simulink model "kepler_basic_2021b"  (R2021b)
settings: Solver=ode4  StartTime=0.0  StopTime=6000  FixedStep=0.01  RelTol=1e-3
(part 1 of 2)
settings Model: Creator=sakur  LastModifiedBy=sakur
settings DebuggingCC: UnconnectedInputMsg=none  UnconnectedOutputMsg=none  UnconnectedLineMsg=none
settings RTWCC: DLArmComputeVersion=20.02.1

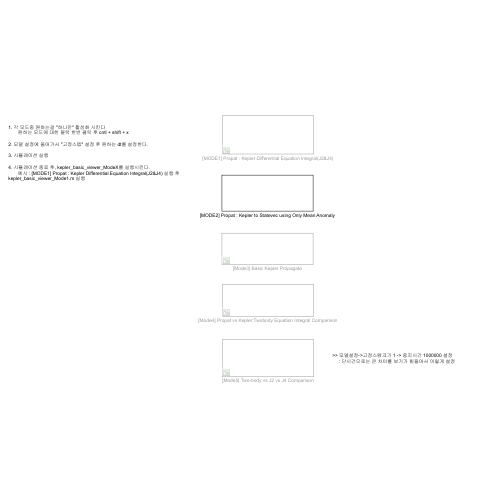
[thumbnail: Simulink's stored preview of the top-level diagram]
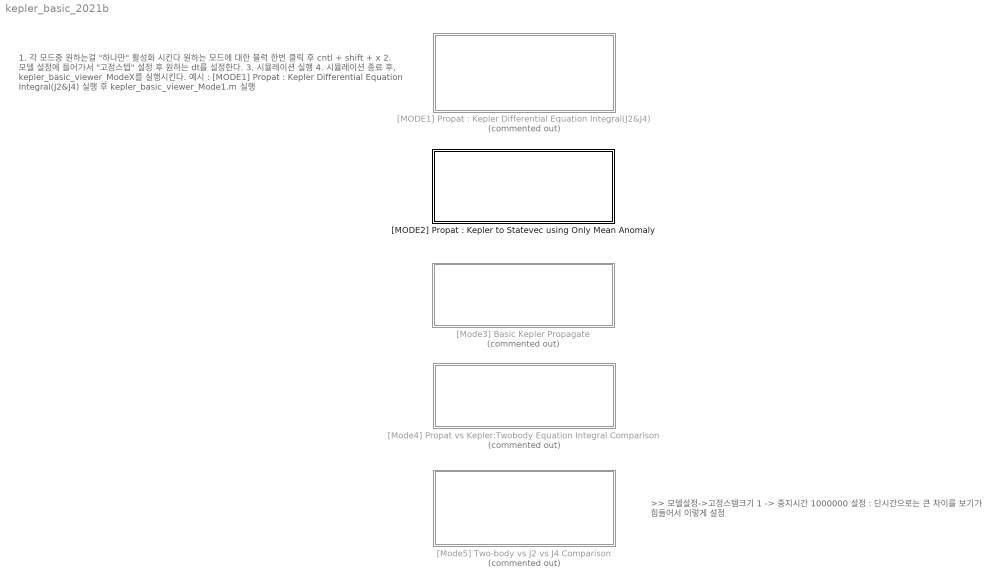
== system kepler_basic_2021b ==
  note: >> 모델설정->고정스템크기 1 -> 중지시간 1000000 설정
      |      : 단시간으로는 큰 차이를 보기가 힘들어서 이렇게 설정
  note: 1. 각 모드중 원하는걸 "하나만" 활성화 시킨다
      | 	원하는 모드에 대한 블럭 한번 클릭 후 cntl + shift + x
      |
      | 2. 모델 설정에 들어가서 "고정스텝" 설정 후 원하는 dt를 설정한다.
      |
      | 3. 시뮬레이션 실행
      |
      | 4. 시뮬레이션 종료 후, kepler_basic_viewer_ModeX를 실행시킨다.
      | 	예시 : [MODE1] Propat : Kepler Differential Equation Integral(J2&J4) 실행 후 kepler_basic_viewer_Mode1.m 실행
  "[MODE1] Propat : Kepler Differential Equation Integral(J2&J4)" : Subsystem  Commented=on
  "[MODE2] Propat : Kepler to Statevec using Only Mean Anomaly" : Subsystem
  "[Mode3] Basic Kepler Propagate" : Subsystem  Commented=on
  "[Mode4] Propat vs Kepler:Twobody Equation Integral Comparison" : Subsystem  Commented=on
  "[Mode5] Two-body vs J2 vs J4 Comparison" : Subsystem  Commented=on

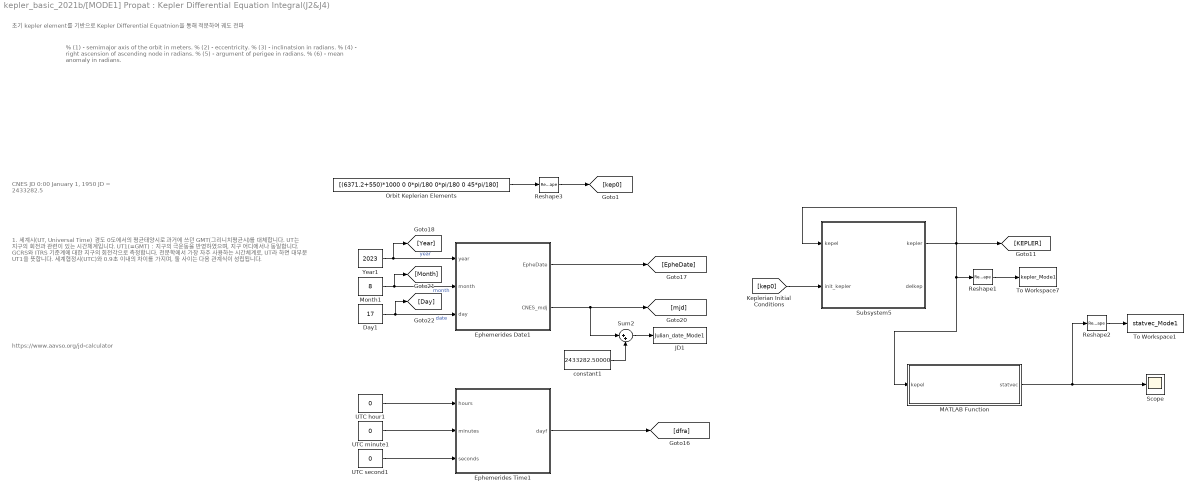
== system kepler_basic_2021b/[MODE1] Propat : Kepler Differential Equation Integral(J2&J4) ==
  note: 초기 kepler element를 기반으로 Kepler Differential Equatnion을 통해 적분하여 궤도 전파
  note: CNES JD
      | 0:00 January 1, 1950
      | JD − 2433282.5
  note: https://www.aavso.org/jd-calculator
  note: 1. 세계시(UT, Universal Time)
      | 경도 0도에서의 평균태양시로 과거에 쓰던 GMT(그리니치평균시)를 대체합니다. UT는 지구의 회전과 관련이 있는 시간체계입니다.
      |
      | UT1(=GMT) : 지구의 극운동을 반영하였으며, 지구 어디에서나 동일합니다. GCRS와 ITRS 기준계에 대한 지구의 회전각으로 측정합니다. 천문학에서 가장 자주 사용하는 시간체계로, UT라 하면 대부분 UT1을 뜻합니다. 세계협정시(UTC)와 0.9초 이내의 차이를 가지며, 둘 사이는 다음 관계식이 성립됩니다.
  note: % (1) - semimajor axis of the orbit in meters.
      | % (2) - eccentricity.
      | % (3) - inclinatsion in radians.
      | % (4) - right ascension of ascending node in radians.
      | % (5) - argument of perigee in radians.
      | % (6) - mean anomaly in radians.
  Day1 : Constant  Value=17
  Ephemerides Date1 : Subsystem
  Ephemerides Time1 : MATLAB Function  TreatAsAtomicUnit=on
  JD1 : ToWorkspace  VariableName=Julian_date_Mode1  SampleTime=-1
  MATLAB Function : MATLAB Function  TreatAsAtomicUnit=on
  Month1 : Constant  Value=8
  Orbit Keplerian Elements : Constant  Value=[(6371.2+550)*1000 0 0*pi/180 0*pi/180 0 45*pi/180]
  Reshape1 : Reshape  OutputDimensionality=Row vector (2-D)
  Reshape2 : Reshape  OutputDimensionality=Row vector (2-D)
  Reshape3 : Reshape  OutputDimensionality=Row vector (2-D)
  Scope : Scope
  Subsystem5 : Subsystem
  Sum2 : Sum  Inputs=|++
  To Workspace1 : ToWorkspace  VariableName=statvec_Mode1  SampleTime=-1
      settings: Save2DSignal=2-D array (concatenate along first dimension)
  To Workspace7 : ToWorkspace  VariableName=kepler_Mode1  SampleTime=-1
      settings: Save2DSignal=2-D array (concatenate along first dimension)
  UTC hour1 : Constant  Value=0
  UTC minute1 : Constant  Value=0
  UTC second1 : Constant  Value=0
  Year1 : Constant  Value=2023
  constant1 : Constant  Value=2433282.50000
  wires:
  Reshape3/1 -> [kep0]
  Year1/1 -> Ephemerides Date1/1(year), [Year]  "year"
  Subsystem5/1(kepler) -> Subsystem5/1(kepel), [KEPLER], Reshape1/1, MATLAB Function/1(kepel)
  Month1/1 -> [Month], Ephemerides Date1/2(month)  "month"
  UTC hour1/1 -> Ephemerides Time1/1(hours)
  Reshape1/1 -> To Workspace7/1
  UTC minute1/1 -> Ephemerides Time1/2(minutes)
  Orbit Keplerian Elements/1 -> Reshape3/1
  MATLAB Function/1(statvec) -> Reshape2/1, Scope/1
  constant1/1 -> Sum2/2
  Day1/1 -> [Day], Ephemerides Date1/3(day)  "date"
  Ephemerides Time1/1(dayf) -> [dfra]
  Ephemerides Date1/2(CNES_mdj) -> Sum2/1, [mjd]
  Ephemerides Date1/1(EpheDate) -> [EpheDate]
  Sum2/1 -> JD1/1
  UTC second1/1 -> Ephemerides Time1/3(seconds)
  [kep0] -> Subsystem5/2(init_kepler)
  Reshape2/1 -> To Workspace1/1

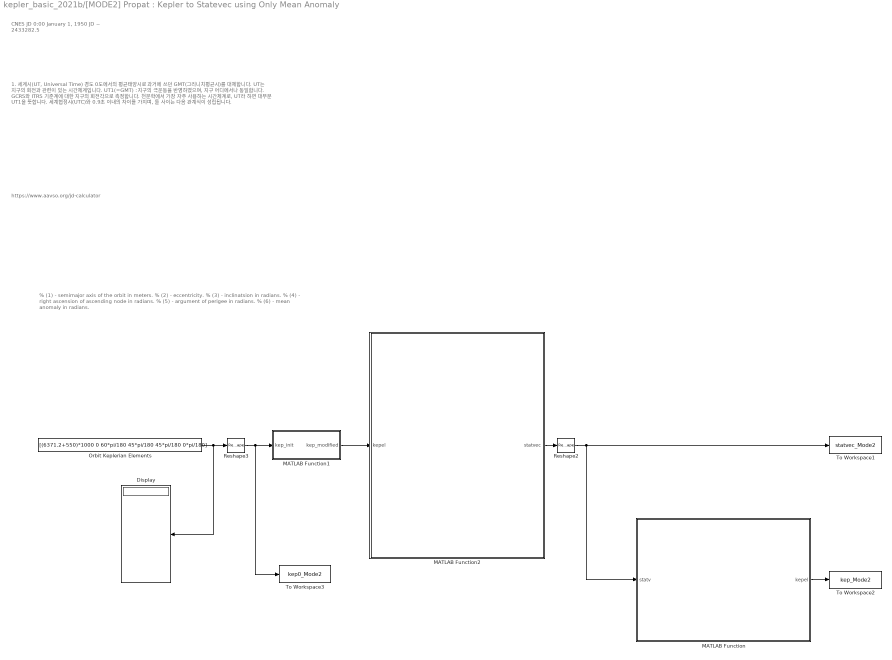
== system kepler_basic_2021b/[MODE2] Propat : Kepler to Statevec using Only Mean Anomaly ==
  note: https://www.aavso.org/jd-calculator
  note: CNES JD
      | 0:00 January 1, 1950
      | JD − 2433282.5
  note: % (1) - semimajor axis of the orbit in meters.
      | % (2) - eccentricity.
      | % (3) - inclinatsion in radians.
      | % (4) - right ascension of ascending node in radians.
      | % (5) - argument of perigee in radians.
      | % (6) - mean anomaly in radians.
  note: 1. 세계시(UT, Universal Time)
      | 경도 0도에서의 평균태양시로 과거에 쓰던 GMT(그리니치평균시)를 대체합니다. UT는 지구의 회전과 관련이 있는 시간체계입니다.
      |
      | UT1(=GMT) : 지구의 극운동을 반영하였으며, 지구 어디에서나 동일합니다. GCRS와 ITRS 기준계에 대한 지구의 회전각으로 측정합니다. 천문학에서 가장 자주 사용하는 시간체계로, UT라 하면 대부분 UT1을 뜻합니다. 세계협정시(UTC)와 0.9초 이내의 차이를 가지며, 둘 사이는 다음 관계식이 성립됩니다.
  Display : Display
  MATLAB Function : MATLAB Function  TreatAsAtomicUnit=on
  MATLAB Function1 : MATLAB Function  TreatAsAtomicUnit=on
  MATLAB Function2 : MATLAB Function  TreatAsAtomicUnit=on
  Orbit Keplerian Elements : Constant  Value=[(6371.2+550)*1000 0 60*pi/180 45*pi/180 45*pi/180 0*pi/180]
  Reshape2 : Reshape  OutputDimensionality=Row vector (2-D)
  Reshape3 : Reshape  OutputDimensionality=Row vector (2-D)
  To Workspace1 : ToWorkspace  VariableName=statvec_Mode2  SampleTime=-1
      settings: Save2DSignal=2-D array (concatenate along first dimension)
  To Workspace2 : ToWorkspace  VariableName=kep_Mode2  SampleTime=-1
      settings: Save2DSignal=2-D array (concatenate along first dimension)
  To Workspace3 : ToWorkspace  VariableName=kep0_Mode2  SampleTime=-1
      settings: Save2DSignal=2-D array (concatenate along first dimension)
  wires:
  Reshape3/1 -> To Workspace3/1, MATLAB Function1/1(kep_init)
  MATLAB Function1/1(kep_modified) -> MATLAB Function2/1(kepel)
  MATLAB Function2/1(statvec) -> Reshape2/1
  Orbit Keplerian Elements/1 -> Display/1, Reshape3/1
  Reshape2/1 -> MATLAB Function/1(statv), To Workspace1/1
  MATLAB Function/1(kepel) -> To Workspace2/1

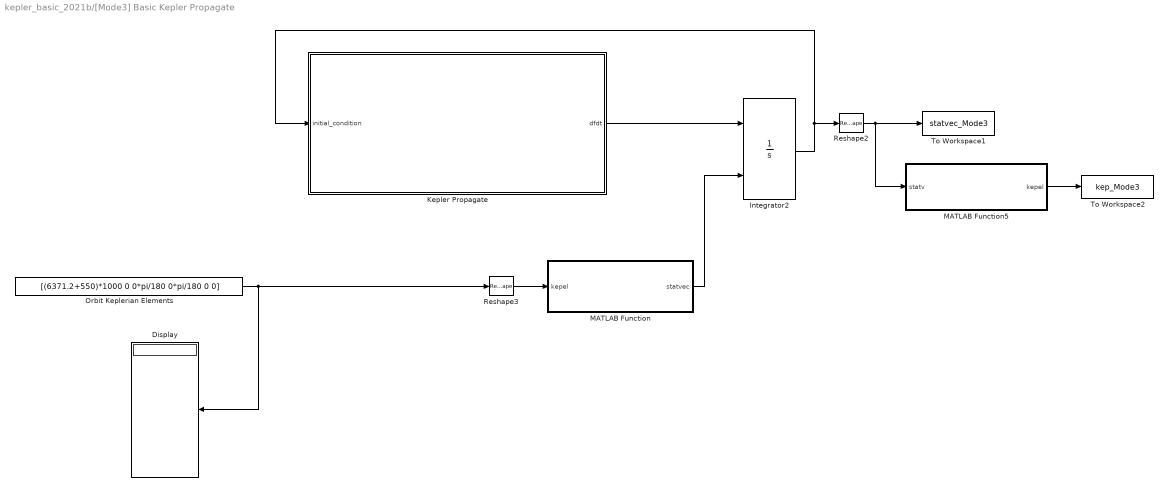
== system kepler_basic_2021b/[Mode3] Basic Kepler Propagate ==
  Display : Display
  Integrator2 : Integrator  InitialConditionSource=external  InitialCondition=[-7000 0 0 0 -9.175045 0 5233.5]'
  Kepler Propagate : MATLAB Function  TreatAsAtomicUnit=on
  MATLAB Function : MATLAB Function  TreatAsAtomicUnit=on
  MATLAB Function5 : MATLAB Function  TreatAsAtomicUnit=on
  Orbit Keplerian Elements : Constant  Value=[(6371.2+550)*1000 0 0*pi/180 0*pi/180 0 0]
  Reshape2 : Reshape  OutputDimensionality=Row vector (2-D)
  Reshape3 : Reshape  OutputDimensionality=Row vector (2-D)
  To Workspace1 : ToWorkspace  VariableName=statvec_Mode3  SampleTime=-1
      settings: Save2DSignal=2-D array (concatenate along first dimension)
  To Workspace2 : ToWorkspace  VariableName=kep_Mode3  SampleTime=-1
      settings: Save2DSignal=2-D array (concatenate along first dimension)
  wires:
  MATLAB Function/1(statvec) -> Integrator2/2
  Kepler Propagate/1(dfdt) -> Integrator2/1
  Reshape2/1 -> MATLAB Function5/1(statv), To Workspace1/1
  Reshape3/1 -> MATLAB Function/1(kepel)
  Orbit Keplerian Elements/1 -> Display/1, Reshape3/1
  Integrator2/1 -> Reshape2/1, Kepler Propagate/1(initial_condition)
  MATLAB Function5/1(kepel) -> To Workspace2/1

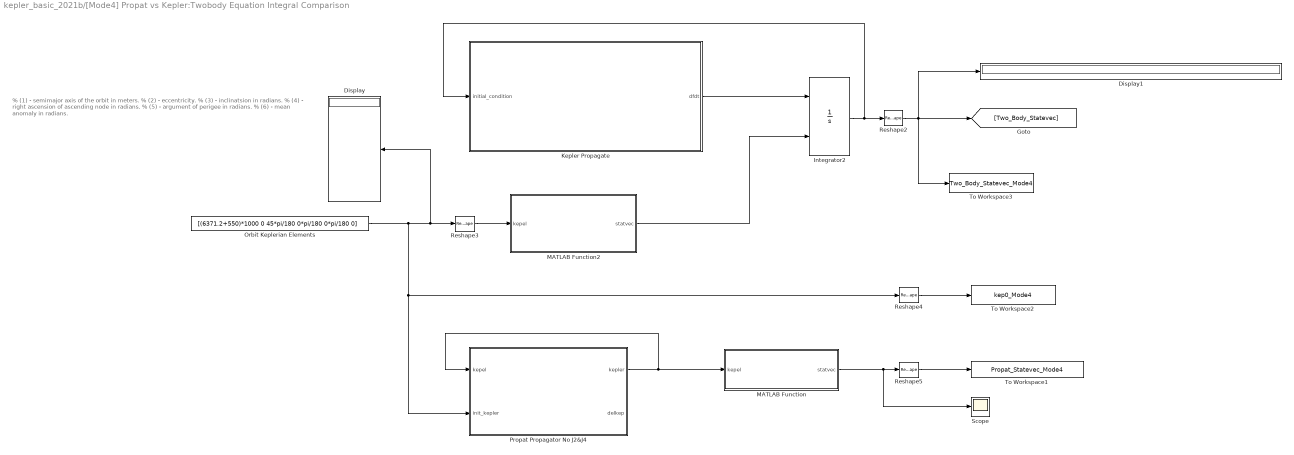
== system kepler_basic_2021b/[Mode4] Propat vs Kepler:Twobody Equation Integral Comparison ==
  note: %		(1) - semimajor axis of the orbit in meters.
      | %		(2) - eccentricity.
      | %		(3) - inclinatsion in radians.
      | %		(4) - right ascension of ascending node in radians.
      | %		(5) - argument of perigee in radians.
      | %		(6) - mean anomaly in radians.
  Display : Display
  Display1 : Display
  Integrator2 : Integrator  InitialConditionSource=external  InitialCondition=[-7000 0 0 0 -9.175045 0 5233.5]'
  Kepler Propagate : MATLAB Function  TreatAsAtomicUnit=on
  MATLAB Function : MATLAB Function  TreatAsAtomicUnit=on
  MATLAB Function2 : MATLAB Function  TreatAsAtomicUnit=on
  Orbit Keplerian Elements : Constant  Value=[(6371.2+550)*1000 0 45*pi/180 0*pi/180 0*pi/180 0]
  Propat Propagator No J2&J4 : Subsystem
  Reshape{2..5} (4 alike) : Reshape  OutputDimensionality=Row vector (2-D)
  Scope : Scope
  To Workspace1 : ToWorkspace  VariableName=Propat_Statevec_Mode4  SampleTime=-1
      settings: Save2DSignal=2-D array (concatenate along first dimension)
  To Workspace2 : ToWorkspace  VariableName=kep0_Mode4  SampleTime=-1
      settings: Save2DSignal=2-D array (concatenate along first dimension)
  To Workspace3 : ToWorkspace  VariableName=Two_Body_Statevec_Mode4  SampleTime=-1
      settings: Save2DSignal=2-D array (concatenate along first dimension)
  wires:
  Integrator2/1 -> Kepler Propagate/1(initial_condition), Reshape2/1
  Reshape3/1 -> MATLAB Function2/1(kepel)
  Reshape5/1 -> To Workspace1/1
  Kepler Propagate/1(dfdt) -> Integrator2/1
  MATLAB Function2/1(statvec) -> Integrator2/2
  Propat Propagator No J2&J4/1(kepler) -> Propat Propagator No J2&J4/1(kepel), MATLAB Function/1(kepel)
  Orbit Keplerian Elements/1 -> Reshape4/1, Propat Propagator No J2&J4/2(init_kepler), Display/1, Reshape3/1
  MATLAB Function/1(statvec) -> Scope/1, Reshape5/1
  Reshape2/1 -> To Workspace3/1, Display1/1, [Two_Body_Statevec]
  Reshape4/1 -> To Workspace2/1

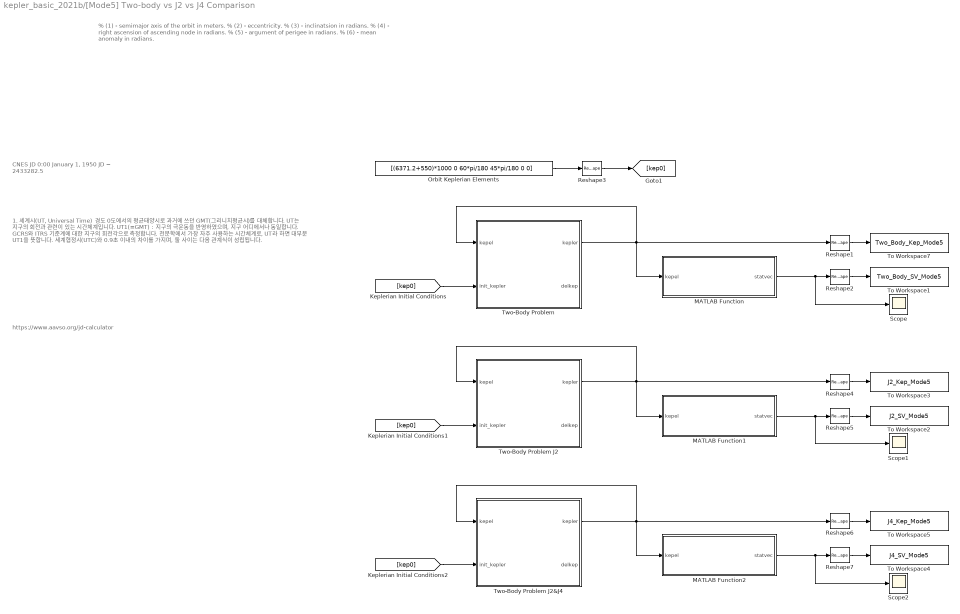
== system kepler_basic_2021b/[Mode5] Two-body vs J2 vs J4 Comparison ==
  note: 1. 세계시(UT, Universal Time)
      | 경도 0도에서의 평균태양시로 과거에 쓰던 GMT(그리니치평균시)를 대체합니다. UT는 지구의 회전과 관련이 있는 시간체계입니다.
      |
      | UT1(=GMT) : 지구의 극운동을 반영하였으며, 지구 어디에서나 동일합니다. GCRS와 ITRS 기준계에 대한 지구의 회전각으로 측정합니다. 천문학에서 가장 자주 사용하는 시간체계로, UT라 하면 대부분 UT1을 뜻합니다. 세계협정시(UTC)와 0.9초 이내의 차이를 가지며, 둘 사이는 다음 관계식이 성립됩니다.
  note: https://www.aavso.org/jd-calculator
  note: CNES JD
      | 0:00 January 1, 1950
      | JD − 2433282.5
  note: % (1) - semimajor axis of the orbit in meters.
      | % (2) - eccentricity.
      | % (3) - inclinatsion in radians.
      | % (4) - right ascension of ascending node in radians.
      | % (5) - argument of perigee in radians.
      | % (6) - mean anomaly in radians.
  MATLAB Function : MATLAB Function  TreatAsAtomicUnit=on
  MATLAB Function1 : MATLAB Function  TreatAsAtomicUnit=on
  MATLAB Function2 : MATLAB Function  TreatAsAtomicUnit=on
  Orbit Keplerian Elements : Constant  Value=[(6371.2+550)*1000 0 60*pi/180 45*pi/180 0 0]
  Reshape{1..7} (7 alike) : Reshape  OutputDimensionality=Row vector (2-D)
  Scope : Scope
  Scope1 : Scope
  Scope2 : Scope
  To Workspace1 : ToWorkspace  VariableName=Two_Body_SV_Mode5  SampleTime=-1
      settings: Save2DSignal=2-D array (concatenate along first dimension)
  To Workspace2 : ToWorkspace  VariableName=J2_SV_Mode5  SampleTime=-1
      settings: Save2DSignal=2-D array (concatenate along first dimension)
  To Workspace3 : ToWorkspace  VariableName=J2_Kep_Mode5  SampleTime=-1
      settings: Save2DSignal=2-D array (concatenate along first dimension)
  To Workspace4 : ToWorkspace  VariableName=J4_SV_Mode5  SampleTime=-1
      settings: Save2DSignal=2-D array (concatenate along first dimension)
  To Workspace5 : ToWorkspace  VariableName=J4_Kep_Mode5  SampleTime=-1
      settings: Save2DSignal=2-D array (concatenate along first dimension)
  To Workspace7 : ToWorkspace  VariableName=Two_Body_Kep_Mode5  SampleTime=-1
      settings: Save2DSignal=2-D array (concatenate along first dimension)
  Two-Body Problem : Subsystem
  Two-Body Problem J2 : Subsystem
  Two-Body Problem J2&J4 : Subsystem
  wires:
  Reshape7/1 -> To Workspace4/1
  Two-Body Problem J2/1(kepler) -> Two-Body Problem J2/1(kepel), Reshape4/1, MATLAB Function1/1(kepel)
  [kep0] -> Two-Body Problem J2/2(init_kepler)
  MATLAB Function1/1(statvec) -> Scope1/1, Reshape5/1
  Reshape4/1 -> To Workspace3/1
  Two-Body Problem/1(kepler) -> Two-Body Problem/1(kepel), Reshape1/1, MATLAB Function/1(kepel)
  Reshape5/1 -> To Workspace2/1
  [kep0] -> Two-Body Problem/2(init_kepler)
  Reshape3/1 -> [kep0]
  MATLAB Function2/1(statvec) -> Scope2/1, Reshape7/1
  Reshape1/1 -> To Workspace7/1
  Reshape2/1 -> To Workspace1/1
  MATLAB Function/1(statvec) -> Scope/1, Reshape2/1
  Two-Body Problem J2&J4/1(kepler) -> Two-Body Problem J2&J4/1(kepel), Reshape6/1, MATLAB Function2/1(kepel)
  Orbit Keplerian Elements/1 -> Reshape3/1
  Reshape6/1 -> To Workspace5/1
  [kep0] -> Two-Body Problem J2&J4/2(init_kepler)

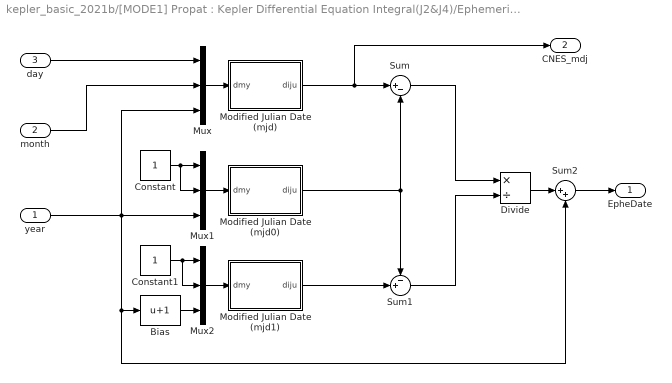
== system kepler_basic_2021b/[MODE1] Propat : Kepler Differential Equation Integral(J2&J4)/Ephemerides Date1 ==
  year : Inport
  month : Inport  Port=2
  day : Inport  Port=3
  Bias : Bias  Bias=1
  Constant : Constant
  Constant1 : Constant
  Divide : Product  Inputs=*/
  Modified Julian Date (mjd) : MATLAB Function  TreatAsAtomicUnit=on
  Modified Julian Date (mjd0) : MATLAB Function  TreatAsAtomicUnit=on
  Modified Julian Date (mjd1) : MATLAB Function  TreatAsAtomicUnit=on
  Mux : Mux  Inputs=3
  Mux1 : Mux  Inputs=3
  Mux2 : Mux  Inputs=3
  Sum : Sum  Inputs=|+-
  Sum1 : Sum  Inputs=-+|
  Sum2 : Sum  Inputs=|++
  EpheDate : Outport
  CNES_mdj : Outport  Port=2
  wires:
  Sum1/1 -> Divide/2
  Modified Julian Date (mjd1)/1(diju) -> Sum1/2
  month/1 -> Mux/2
  year/1 -> Mux1/3, Mux/3, Bias/1, Sum2/2
  Mux1/1 -> Modified Julian Date (mjd0)/1(dmy)
  day/1 -> Mux/1
  Mux/1 -> Modified Julian Date (mjd)/1(dmy)
  Mux2/1 -> Modified Julian Date (mjd1)/1(dmy)
  Bias/1 -> Mux2/3
  Modified Julian Date (mjd)/1(diju) -> CNES_mdj/1, Sum/1
  Constant1/1 -> Mux2/2, Mux2/1
  Sum/1 -> Divide/1
  Constant/1 -> Mux1/2, Mux1/1
  Modified Julian Date (mjd0)/1(diju) -> Sum1/1, Sum/2
  Divide/1 -> Sum2/1
  Sum2/1 -> EpheDate/1

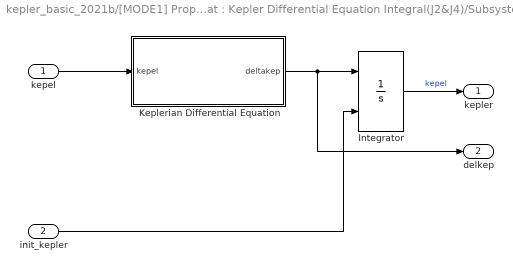
== system kepler_basic_2021b/[MODE1] Propat : Kepler Differential Equation Integral(J2&J4)/Subsystem5 ==
  kepel : Inport
  init_kepler : Inport  Port=2
  Integrator : Integrator  InitialConditionSource=external
  Keplerian Differential Equation : MATLAB Function  TreatAsAtomicUnit=on
  kepler : Outport
  delkep : Outport  Port=2
  wires:
  Integrator/1 -> kepler/1  "kepel"
  Keplerian Differential Equation/1(deltakep) -> delkep/1, Integrator/1
  init_kepler/1 -> Integrator/2
  kepel/1 -> Keplerian Differential Equation/1(kepel)

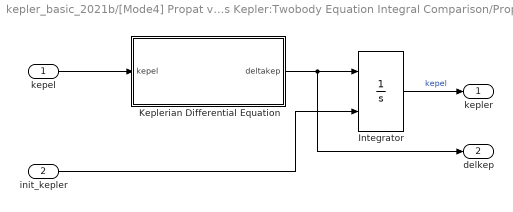
== system kepler_basic_2021b/[Mode4] Propat vs Kepler:Twobody Equation Integral Comparison/Propat Propagator No J2&J4 ==
  kepel : Inport
  init_kepler : Inport  Port=2
  Integrator : Integrator  InitialConditionSource=external
  Keplerian Differential Equation : MATLAB Function  TreatAsAtomicUnit=on
  kepler : Outport
  delkep : Outport  Port=2
  wires:
  Integrator/1 -> kepler/1  "kepel"
  Keplerian Differential Equation/1(deltakep) -> delkep/1, Integrator/1
  init_kepler/1 -> Integrator/2
  kepel/1 -> Keplerian Differential Equation/1(kepel)

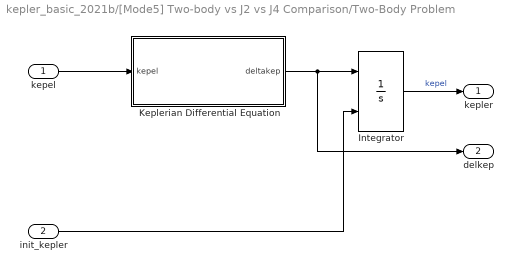
== system kepler_basic_2021b/[Mode5] Two-body vs J2 vs J4 Comparison/Two-Body Problem ==
  kepel : Inport
  init_kepler : Inport  Port=2
  Integrator : Integrator  InitialConditionSource=external
  Keplerian Differential Equation : MATLAB Function  TreatAsAtomicUnit=on
  kepler : Outport
  delkep : Outport  Port=2
  wires:
  Integrator/1 -> kepler/1  "kepel"
  Keplerian Differential Equation/1(deltakep) -> delkep/1, Integrator/1
  init_kepler/1 -> Integrator/2
  kepel/1 -> Keplerian Differential Equation/1(kepel)

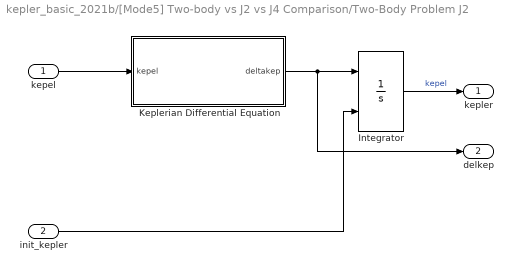
== system kepler_basic_2021b/[Mode5] Two-body vs J2 vs J4 Comparison/Two-Body Problem J2 ==
  kepel : Inport
  init_kepler : Inport  Port=2
  Integrator : Integrator  InitialConditionSource=external
  Keplerian Differential Equation : MATLAB Function  TreatAsAtomicUnit=on
  kepler : Outport
  delkep : Outport  Port=2
  wires:
  Integrator/1 -> kepler/1  "kepel"
  Keplerian Differential Equation/1(deltakep) -> delkep/1, Integrator/1
  init_kepler/1 -> Integrator/2
  kepel/1 -> Keplerian Differential Equation/1(kepel)

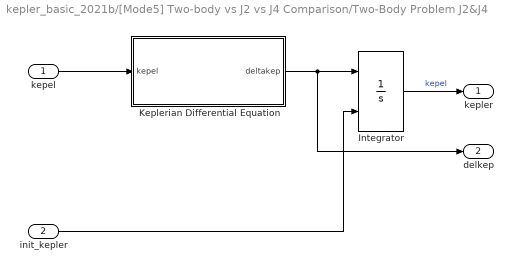
== system kepler_basic_2021b/[Mode5] Two-body vs J2 vs J4 Comparison/Two-Body Problem J2&J4 ==
  kepel : Inport
  init_kepler : Inport  Port=2
  Integrator : Integrator  InitialConditionSource=external
  Keplerian Differential Equation : MATLAB Function  TreatAsAtomicUnit=on
  kepler : Outport
  delkep : Outport  Port=2
  wires:
  Integrator/1 -> kepler/1  "kepel"
  Keplerian Differential Equation/1(deltakep) -> delkep/1, Integrator/1
  init_kepler/1 -> Integrator/2
  kepel/1 -> Keplerian Differential Equation/1(kepel)

== matlab function kepler_basic_2021b/[Mode5] Two-body vs J2 vs J4 Comparison/MATLAB Function1 ==
  data: kepel input; statvec output
function statvec  = kepel_statvec (kepel)
%  [statvec] = kepel_statvec (kepel)
%	The function kepel_statvec transforms the keplerian
%	elements kepel into the corresponding state vector in
%	the same reference system.
%
% Input:
%	kepel
% 		vector containing the keplerian elements:
%		(1) - semimajor axis of the orbit in meters.
%		(2) - eccentricity.
%		(3) - inclinatsion in radians.
%		(4) - right ascension of ascending node in radians.
%		(5) - argument of perigee in radians.
%		(6) - mean anomaly in radians.
% Output:
%	statvec
%  		state vector in meters and meters/second.
%
% Authors:
%	Helio K. Kuga;
%	Valder M. Medeiros;
%	Valdemir Carrara		february/80		version 1.0
%	Valdemir Carrara		july 2005		(C version)
%   Valdemir Carrara            March/09        Matlab

EARTH_GRAVITY	= 3.9860064e+14;		% Earth's gravitational constant (m**3/s**2)

a    = kepel(1);	% semi-major axis
exc  = kepel(2);	% eccentricity

c1   = sqrt(1. - exc*exc);

%     rotation matrix

orb2iner = rotmaz(-kepel(4))*rotmax(-kepel(3))*rotmaz(-kepel(5));

%     Kepler's equation

E    = kepler(kepel(6), exc);

sE   = sin(E);
cE   = cos(E);
c3   = sqrt(EARTH_GRAVITY/a)/(1. - exc*cE);

%     state vector

statvec = [[a*(cE - exc), a*c1*sE, 0]*orb2iner', [-c3*sE, c1*c3*cE, 0]*orb2iner'];

end

function [rot_mat] = rotmax (angle)
% [rot_mat] = rotmax (angle)
%   To obtain the rotation matrix around the X axis given the
%   rotation angle.
% inputs:
%   angle
%       rotation angle, in radians.
% outputs:
%   rot_mat
%       rotation matrix (3, 3)
%

% Valdemir Carrara, Sep, 1998

coan    =  cos(angle);
sian    =  sin(angle);

rot_mat =  [1, 0, 0; 0, coan, sian; 0, -sian, coan];

end

function [rot_mat] = rotmay (angle)
% [rot_mat] = rotmay (angle)
%   To obtain the rotation matrix around the Y axis given the
%   rotation angle.
% inputs:
%   angle
%       rotation angle, in radians.
% outputs:
%   rot_mat
%       rotation matrix (3, 3)
%

% Valdemir Carrara, Sep, 1998


coan    =  cos(angle);
sian    =  sin(angle);

rot_mat =  [coan, 0, -sian; 0, 1, 0; sian, 0, coan];

end

function [rot_mat] = rotmaz (angle)
% [rot_mat] = rotmaz (angle)
%   To obtain the rotation matrix around the Z axis given the
%   rotation angle.
% inputs:
%   angle
%       rotation angle, in radians.
% outputs:
%   rot_mat
%       rotation matrix (3, 3)
%

% Valdemir Carrara, Sep, 1998

coan    =  cos(angle);
sian    =  sin(angle);

rot_mat =  [coan, sian, 0; -sian, coan, 0; 0, 0, 1];
end

function [eccentric] = kepler (mean_anomaly, eccentricity)
% [eccentric] = kepler (mean_anomaly, eccentricity)
%	The subroutine kepler finds a solution to the
%	kepler's equation.
%
% Input:
%	mean_anomaly
%		mean anomaly in radians.
%	eccentricity
%		eccentricity.
%
% Output:
%	eccentric
%		eccentric anomaly in radians.
%
% Authors:
%	Valder M. de Medeiros		june/81		version 2.0
%	Valdemir Carrara			july 2005	(C version)
%   Valdemir Carrara            March/09        Matlab

exc2    = eccentricity*eccentricity;
am1     = mod (mean_anomaly, 2*pi);
am2     = am1 + am1;
am3     = am1 + am2;
shoot   = am1 + eccentricity*(1. - 0.125*exc2)*sin(am1) + ...
		0.5*exc2*(sin(am2) + 0.75*eccentricity*sin(am3));
shoot   = mod (shoot, 2*pi);

e1      = 1.0;
ic      = 0;

while ((abs(e1) > 1.e-12) && (ic <= 10)) 
	e1    = (shoot - am1 - eccentricity*sin(shoot)) / ...
			(1.0 - eccentricity*cos(shoot));
    shoot = shoot - e1;
    ic    = ic + 1;
end

if (ic >= 10)
    disp ('warning ** subroutine kepler did not converge in 10 iterations');
end

eccentric = shoot;


end

== matlab function kepler_basic_2021b/[Mode5] Two-body vs J2 vs J4 Comparison/Two-Body Problem J2/Keplerian Differential Equation ==
  data: kepel input; deltakep output
function deltakep  = delkep(kepel)
% [deltakep] = delkep (kep_el)
%	Function delkep calculates the rate of
%	variation of keplerian elements, considering only
%	J2 and J4.
%
% Input:
%	kep_el
% 		vector with the keplerian elements:
%		(1) - semimajor axis of the orbit in meters.
%		(2) - eccentricity.
%		(3) - inclination in radians.
%		(4) - right ascension of ascending node in radians.
%		(5) - argument of perigee in radians.
%		(6) - mean anomaly in radians.
%       Obs: 4,5 and 6 are not used
%
% Output:
%	deltakep
%		(1) = 0
%		(2) = 0
%		(3) = 0
%		(4) - variation rate of the right ascension of
%		      ascending node, in radians/second.
%		(5) - variation rate of the argument of perigee,
%			  in radians/second.
%		(6) - variation rate of the mean anomaly, in
%			  radians/second.
%
% Authors:
%	Valder M. de Medeiros  	september/81 	version 1.0
%	Valdemir Carrara 		july 2005		(C Version)
%   Valdemir Carrara            March/09        Matlab

EARTH_RADIUS	= 6378139.;				% Earth's radius in meters
EARTH_GRAVITY	= 3.9860064e+14;		% Earth's gravitational constant (m**3/s**2)
J_2 			=  1.0826268362e-3;		% = 484.16544e-6 * SQRT(5.e0)
% J_4 			= -1.62336e-6;			% = -0.54112e-6 * 3e0
% J_2 			=  0;		% = 484.16544e-6 * SQRT(5.e0)
J_4 			=  0;			% = -0.54112e-6 * 3e0

seix = kepel(1);
exce = kepel(2);
exc2 = exce*exce;
eta2 = 1. - exc2;
eta1 = sqrt(eta2);
teta = cos(kepel(3));
tet2 = teta*teta;
tet4 = tet2*tet2;
aux0 = sqrt(EARTH_GRAVITY/(seix*seix*seix));
plar = EARTH_RADIUS/(seix*eta2);
pla2 = plar*plar;
gam2 = 0.5*J_2*pla2;
gam4 = -0.375*J_4*pla2*pla2;

deltakep = [0, 0, 0, 0, 0, 0];

deltakep(4) = aux0*teta*(3.*gam2*(-1. + 0.125*gam2*(9.*eta2 + 12.*eta1 - ...
	   5. - (5.*eta2 + 36.*eta1 + 35.)*tet2)) + ...
	   1.25*gam4*(5. - 3.*eta2)*(3. - 7.*tet2));
deltakep(5) = aux0*(1.5*gam2*((5.*tet2 - 1.) + ...
	   0.0625*gam2*(25.*eta2 + 24.*eta1 - ...
	   35. + (90. - 192.*eta1 - 126.*eta2)*tet2 + ...
	   (385. + 360.*eta1 + 45.*eta2)*tet4)) + ...
	   0.3125*gam4*(21. - 9.*eta2 + (-270. + 126.*eta2)*tet2 + ...
	   (385. - 189.*eta2)*tet4));
deltakep(6) = aux0*(1. + eta1*(1.5*gam2*((3.*tet2 - 1.) + ...
	   0.0625*gam2*(16.*eta1 + 25.*eta2 - 15. + ...
	   (30. - 96.*eta1 - 90.*eta2)*tet2 + ...
	   (105. + 144.*eta1 + 25.*eta2)*tet4)) + ...
	   0.9375*gam4*exc2*(3. - 30.*tet2 + 35.*tet4)));

end

== matlab function kepler_basic_2021b/[Mode5] Two-body vs J2 vs J4 Comparison/MATLAB Function2 ==
  data: kepel input; statvec output
function statvec  = kepel_statvec (kepel)
%  [statvec] = kepel_statvec (kepel)
%	The function kepel_statvec transforms the keplerian
%	elements kepel into the corresponding state vector in
%	the same reference system.
%
% Input:
%	kepel
% 		vector containing the keplerian elements:
%		(1) - semimajor axis of the orbit in meters.
%		(2) - eccentricity.
%		(3) - inclinatsion in radians.
%		(4) - right ascension of ascending node in radians.
%		(5) - argument of perigee in radians.
%		(6) - mean anomaly in radians.
% Output:
%	statvec
%  		state vector in meters and meters/second.
%
% Authors:
%	Helio K. Kuga;
%	Valder M. Medeiros;
%	Valdemir Carrara		february/80		version 1.0
%	Valdemir Carrara		july 2005		(C version)
%   Valdemir Carrara            March/09        Matlab

EARTH_GRAVITY	= 3.9860064e+14;		% Earth's gravitational constant (m**3/s**2)

a    = kepel(1);	% semi-major axis
exc  = kepel(2);	% eccentricity

c1   = sqrt(1. - exc*exc);

%     rotation matrix

orb2iner = rotmaz(-kepel(4))*rotmax(-kepel(3))*rotmaz(-kepel(5));

%     Kepler's equation

E    = kepler(kepel(6), exc);

sE   = sin(E);
cE   = cos(E);
c3   = sqrt(EARTH_GRAVITY/a)/(1. - exc*cE);

%     state vector

statvec = [[a*(cE - exc), a*c1*sE, 0]*orb2iner', [-c3*sE, c1*c3*cE, 0]*orb2iner'];

end

function [rot_mat] = rotmax (angle)
% [rot_mat] = rotmax (angle)
%   To obtain the rotation matrix around the X axis given the
%   rotation angle.
% inputs:
%   angle
%       rotation angle, in radians.
% outputs:
%   rot_mat
%       rotation matrix (3, 3)
%

% Valdemir Carrara, Sep, 1998

coan    =  cos(angle);
sian    =  sin(angle);

rot_mat =  [1, 0, 0; 0, coan, sian; 0, -sian, coan];

end

function [rot_mat] = rotmay (angle)
% [rot_mat] = rotmay (angle)
%   To obtain the rotation matrix around the Y axis given the
%   rotation angle.
% inputs:
%   angle
%       rotation angle, in radians.
% outputs:
%   rot_mat
%       rotation matrix (3, 3)
%

% Valdemir Carrara, Sep, 1998


coan    =  cos(angle);
sian    =  sin(angle);

rot_mat =  [coan, 0, -sian; 0, 1, 0; sian, 0, coan];

end

function [rot_mat] = rotmaz (angle)
% [rot_mat] = rotmaz (angle)
%   To obtain the rotation matrix around the Z axis given the
%   rotation angle.
% inputs:
%   angle
%       rotation angle, in radians.
% outputs:
%   rot_mat
%       rotation matrix (3, 3)
%

% Valdemir Carrara, Sep, 1998

coan    =  cos(angle);
sian    =  sin(angle);

rot_mat =  [coan, sian, 0; -sian, coan, 0; 0, 0, 1];
end

function [eccentric] = kepler (mean_anomaly, eccentricity)
% [eccentric] = kepler (mean_anomaly, eccentricity)
%	The subroutine kepler finds a solution to the
%	kepler's equation.
%
% Input:
%	mean_anomaly
%		mean anomaly in radians.
%	eccentricity
%		eccentricity.
%
% Output:
%	eccentric
%		eccentric anomaly in radians.
%
% Authors:
%	Valder M. de Medeiros		june/81		version 2.0
%	Valdemir Carrara			july 2005	(C version)
%   Valdemir Carrara            March/09        Matlab

exc2    = eccentricity*eccentricity;
am1     = mod (mean_anomaly, 2*pi);
am2     = am1 + am1;
am3     = am1 + am2;
shoot   = am1 + eccentricity*(1. - 0.125*exc2)*sin(am1) + ...
		0.5*exc2*(sin(am2) + 0.75*eccentricity*sin(am3));
shoot   = mod (shoot, 2*pi);

e1      = 1.0;
ic      = 0;

while ((abs(e1) > 1.e-12) && (ic <= 10)) 
	e1    = (shoot - am1 - eccentricity*sin(shoot)) / ...
			(1.0 - eccentricity*cos(shoot));
    shoot = shoot - e1;
    ic    = ic + 1;
end

if (ic >= 10)
    disp ('warning ** subroutine kepler did not converge in 10 iterations');
end

eccentric = shoot;


end

== matlab function kepler_basic_2021b/[Mode5] Two-body vs J2 vs J4 Comparison/Two-Body Problem J2&J4/Keplerian Differential Equation ==
  data: kepel input; deltakep output
function deltakep  = delkep(kepel)
% [deltakep] = delkep (kep_el)
%	Function delkep calculates the rate of
%	variation of keplerian elements, considering only
%	J2 and J4.
%
% Input:
%	kep_el
% 		vector with the keplerian elements:
%		(1) - semimajor axis of the orbit in meters.
%		(2) - eccentricity.
%		(3) - inclination in radians.
%		(4) - right ascension of ascending node in radians.
%		(5) - argument of perigee in radians.
%		(6) - mean anomaly in radians.
%       Obs: 4,5 and 6 are not used
%
% Output:
%	deltakep
%		(1) = 0
%		(2) = 0
%		(3) = 0
%		(4) - variation rate of the right ascension of
%		      ascending node, in radians/second.
%		(5) - variation rate of the argument of perigee,
%			  in radians/second.
%		(6) - variation rate of the mean anomaly, in
%			  radians/second.
%
% Authors:
%	Valder M. de Medeiros  	september/81 	version 1.0
%	Valdemir Carrara 		july 2005		(C Version)
%   Valdemir Carrara            March/09        Matlab

EARTH_RADIUS	= 6378139.;				% Earth's radius in meters
EARTH_GRAVITY	= 3.9860064e+14;		% Earth's gravitational constant (m**3/s**2)
J_2 			=  1.0826268362e-3;		% = 484.16544e-6 * SQRT(5.e0)
J_4 			= -1.62336e-6;			% = -0.54112e-6 * 3e0

seix = kepel(1);
exce = kepel(2);
exc2 = exce*exce;
eta2 = 1. - exc2;
eta1 = sqrt(eta2);
teta = cos(kepel(3));
tet2 = teta*teta;
tet4 = tet2*tet2;
aux0 = sqrt(EARTH_GRAVITY/(seix*seix*seix));
plar = EARTH_RADIUS/(seix*eta2);
pla2 = plar*plar;
gam2 = 0.5*J_2*pla2;
gam4 = -0.375*J_4*pla2*pla2;

deltakep = [0, 0, 0, 0, 0, 0];

deltakep(4) = aux0*teta*(3.*gam2*(-1. + 0.125*gam2*(9.*eta2 + 12.*eta1 - ...
	   5. - (5.*eta2 + 36.*eta1 + 35.)*tet2)) + ...
	   1.25*gam4*(5. - 3.*eta2)*(3. - 7.*tet2));
deltakep(5) = aux0*(1.5*gam2*((5.*tet2 - 1.) + ...
	   0.0625*gam2*(25.*eta2 + 24.*eta1 - ...
	   35. + (90. - 192.*eta1 - 126.*eta2)*tet2 + ...
	   (385. + 360.*eta1 + 45.*eta2)*tet4)) + ...
	   0.3125*gam4*(21. - 9.*eta2 + (-270. + 126.*eta2)*tet2 + ...
	   (385. - 189.*eta2)*tet4));
deltakep(6) = aux0*(1. + eta1*(1.5*gam2*((3.*tet2 - 1.) + ...
	   0.0625*gam2*(16.*eta1 + 25.*eta2 - 15. + ...
	   (30. - 96.*eta1 - 90.*eta2)*tet2 + ...
	   (105. + 144.*eta1 + 25.*eta2)*tet4)) + ...
	   0.9375*gam4*exc2*(3. - 30.*tet2 + 35.*tet4)));

end

== matlab function kepler_basic_2021b/[Mode5] Two-body vs J2 vs J4 Comparison/MATLAB Function ==
  data: kepel input; statvec output
function statvec  = kepel_statvec (kepel)
%  [statvec] = kepel_statvec (kepel)
%	The function kepel_statvec transforms the keplerian
%	elements kepel into the corresponding state vector in
%	the same reference system.
%
% Input:
%	kepel
% 		vector containing the keplerian elements:
%		(1) - semimajor axis of the orbit in meters.
%		(2) - eccentricity.
%		(3) - inclinatsion in radians.
%		(4) - right ascension of ascending node in radians.
%		(5) - argument of perigee in radians.
%		(6) - mean anomaly in radians.
% Output:
%	statvec
%  		state vector in meters and meters/second.
%
% Authors:
%	Helio K. Kuga;
%	Valder M. Medeiros;
%	Valdemir Carrara		february/80		version 1.0
%	Valdemir Carrara		july 2005		(C version)
%   Valdemir Carrara            March/09        Matlab

EARTH_GRAVITY	= 3.9860064e+14;		% Earth's gravitational constant (m**3/s**2)

a    = kepel(1);	% semi-major axis
exc  = kepel(2);	% eccentricity

c1   = sqrt(1. - exc*exc);

%     rotation matrix

orb2iner = rotmaz(-kepel(4))*rotmax(-kepel(3))*rotmaz(-kepel(5));

%     Kepler's equation

E    = kepler(kepel(6), exc);

sE   = sin(E);
cE   = cos(E);
c3   = sqrt(EARTH_GRAVITY/a)/(1. - exc*cE);

%     state vector

statvec = [[a*(cE - exc), a*c1*sE, 0]*orb2iner', [-c3*sE, c1*c3*cE, 0]*orb2iner'];

end

function [rot_mat] = rotmax (angle)
% [rot_mat] = rotmax (angle)
%   To obtain the rotation matrix around the X axis given the
%   rotation angle.
% inputs:
%   angle
%       rotation angle, in radians.
% outputs:
%   rot_mat
%       rotation matrix (3, 3)
%

% Valdemir Carrara, Sep, 1998

coan    =  cos(angle);
sian    =  sin(angle);

rot_mat =  [1, 0, 0; 0, coan, sian; 0, -sian, coan];

end

function [rot_mat] = rotmay (angle)
% [rot_mat] = rotmay (angle)
%   To obtain the rotation matrix around the Y axis given the
%   rotation angle.
% inputs:
%   angle
%       rotation angle, in radians.
% outputs:
%   rot_mat
%       rotation matrix (3, 3)
%

% Valdemir Carrara, Sep, 1998


coan    =  cos(angle);
sian    =  sin(angle);

rot_mat =  [coan, 0, -sian; 0, 1, 0; sian, 0, coan];

end

function [rot_mat] = rotmaz (angle)
% [rot_mat] = rotmaz (angle)
%   To obtain the rotation matrix around the Z axis given the
%   rotation angle.
% inputs:
%   angle
%       rotation angle, in radians.
% outputs:
%   rot_mat
%       rotation matrix (3, 3)
%

% Valdemir Carrara, Sep, 1998

coan    =  cos(angle);
sian    =  sin(angle);

rot_mat =  [coan, sian, 0; -sian, coan, 0; 0, 0, 1];
end

function [eccentric] = kepler (mean_anomaly, eccentricity)
% [eccentric] = kepler (mean_anomaly, eccentricity)
%	The subroutine kepler finds a solution to the
%	kepler's equation.
%
% Input:
%	mean_anomaly
%		mean anomaly in radians.
%	eccentricity
%		eccentricity.
%
% Output:
%	eccentric
%		eccentric anomaly in radians.
%
% Authors:
%	Valder M. de Medeiros		june/81		version 2.0
%	Valdemir Carrara			july 2005	(C version)
%   Valdemir Carrara            March/09        Matlab

exc2    = eccentricity*eccentricity;
am1     = mod (mean_anomaly, 2*pi);
am2     = am1 + am1;
am3     = am1 + am2;
shoot   = am1 + eccentricity*(1. - 0.125*exc2)*sin(am1) + ...
		0.5*exc2*(sin(am2) + 0.75*eccentricity*sin(am3));
shoot   = mod (shoot, 2*pi);

e1      = 1.0;
ic      = 0;

while ((abs(e1) > 1.e-12) && (ic <= 10)) 
	e1    = (shoot - am1 - eccentricity*sin(shoot)) / ...
			(1.0 - eccentricity*cos(shoot));
    shoot = shoot - e1;
    ic    = ic + 1;
end

if (ic >= 10)
    disp ('warning ** subroutine kepler did not converge in 10 iterations');
end

eccentric = shoot;


end

== matlab function kepler_basic_2021b/[Mode5] Two-body vs J2 vs J4 Comparison/Two-Body Problem/Keplerian Differential Equation ==
  data: kepel input; deltakep output
function deltakep  = delkep(kepel)
% [deltakep] = delkep (kep_el)
%	Function delkep calculates the rate of
%	variation of keplerian elements, considering only
%	J2 and J4.
%
% Input:
%	kep_el
% 		vector with the keplerian elements:
%		(1) - semimajor axis of the orbit in meters.
%		(2) - eccentricity.
%		(3) - inclination in radians.
%		(4) - right ascension of ascending node in radians.
%		(5) - argument of perigee in radians.
%		(6) - mean anomaly in radians.
%       Obs: 4,5 and 6 are not used
%
% Output:
%	deltakep
%		(1) = 0
%		(2) = 0
%		(3) = 0
%		(4) - variation rate of the right ascension of
%		      ascending node, in radians/second.
%		(5) - variation rate of the argument of perigee,
%			  in radians/second.
%		(6) - variation rate of the mean anomaly, in
%			  radians/second.
%
% Authors:
%	Valder M. de Medeiros  	september/81 	version 1.0
%	Valdemir Carrara 		july 2005		(C Version)
%   Valdemir Carrara            March/09        Matlab

EARTH_RADIUS	= 6378139.;				% Earth's radius in meters
EARTH_GRAVITY	= 3.9860064e+14;		% Earth's gravitational constant (m**3/s**2)
% J_2 			=  1.0826268362e-3;		% = 484.16544e-6 * SQRT(5.e0)
% J_4 			= -1.62336e-6;			% = -0.54112e-6 * 3e0
J_2 			=  0;		% = 484.16544e-6 * SQRT(5.e0)
J_4 			=  0;			% = -0.54112e-6 * 3e0

seix = kepel(1);
exce = kepel(2);
exc2 = exce*exce;
eta2 = 1. - exc2;
eta1 = sqrt(eta2);
teta = cos(kepel(3));
tet2 = teta*teta;
tet4 = tet2*tet2;
aux0 = sqrt(EARTH_GRAVITY/(seix*seix*seix));
plar = EARTH_RADIUS/(seix*eta2);
pla2 = plar*plar;
gam2 = 0.5*J_2*pla2;
gam4 = -0.375*J_4*pla2*pla2;

deltakep = [0, 0, 0, 0, 0, 0];

deltakep(4) = aux0*teta*(3.*gam2*(-1. + 0.125*gam2*(9.*eta2 + 12.*eta1 - ...
	   5. - (5.*eta2 + 36.*eta1 + 35.)*tet2)) + ...
	   1.25*gam4*(5. - 3.*eta2)*(3. - 7.*tet2));
deltakep(5) = aux0*(1.5*gam2*((5.*tet2 - 1.) + ...
	   0.0625*gam2*(25.*eta2 + 24.*eta1 - ...
	   35. + (90. - 192.*eta1 - 126.*eta2)*tet2 + ...
	   (385. + 360.*eta1 + 45.*eta2)*tet4)) + ...
	   0.3125*gam4*(21. - 9.*eta2 + (-270. + 126.*eta2)*tet2 + ...
	   (385. - 189.*eta2)*tet4));
deltakep(6) = aux0*(1. + eta1*(1.5*gam2*((3.*tet2 - 1.) + ...
	   0.0625*gam2*(16.*eta1 + 25.*eta2 - 15. + ...
	   (30. - 96.*eta1 - 90.*eta2)*tet2 + ...
	   (105. + 144.*eta1 + 25.*eta2)*tet4)) + ...
	   0.9375*gam4*exc2*(3. - 30.*tet2 + 35.*tet4)));

end

== matlab function kepler_basic_2021b/[MODE1] Propat : Kepler Differential Equation Integral(J2&J4)/Ephemerides Date1/Modified Julian Date (mjd) ==
  data: dmy input; diju output
function diju  =  djm (dmy)
% [diju] = djm (day, month, year)
%    The function djm furnishes the Modified Julian
%    Date with reference to the day, month and year,
%    at zero hours of the day.
% inputs:
%   dmy(1): day, day of the month
%   dmy(2): month, month of the year
%   dmy(3): year

% outputs:
%   diju
%       Modified Julian Date in days, referred to 1950.0. 
%
% Valdemir Carrara, Apr, 2003
%

diju = 367*dmy(3) + dmy(1) - 712269 + fix(275*dmy(2)/9)- fix(7*(dmy(3)+fix((dmy(2)+9)/12))/4);

== matlab function kepler_basic_2021b/[MODE1] Propat : Kepler Differential Equation Integral(J2&J4)/Ephemerides Date1/Modified Julian Date (mjd0) ==
  data: dmy input; diju output
function diju  =  djm (dmy)
% [diju] = djm (day, month, year)
%    The function djm furnishes the Modified Julian
%    Date with reference to the day, month and year,
%    at zero hours of the day.
% inputs:
%   dmy(1): day, day of the month
%   dmy(2): month, month of the year
%   dmy(3): year

% outputs:
%   diju
%       Modified Julian Date in days, referred to 1950.0. 
%
% Valdemir Carrara, Apr, 2003
%

diju = 367*dmy(3) + dmy(1) - 712269 + fix(275*dmy(2)/9)- fix(7*(dmy(3)+fix((dmy(2)+9)/12))/4);

== matlab function kepler_basic_2021b/[MODE1] Propat : Kepler Differential Equation Integral(J2&J4)/Ephemerides Date1/Modified Julian Date (mjd1) ==
  data: dmy input; diju output
function diju  =  djm (dmy)
% [diju] = djm (day, month, year)
%    The function djm furnishes the Modified Julian
%    Date with reference to the day, month and year,
%    at zero hours of the day.
% inputs:
%   dmy(1): day, day of the month
%   dmy(2): month, month of the year
%   dmy(3): year

% outputs:
%   diju
%       Modified Julian Date in days, referred to 1950.0. 
%
% Valdemir Carrara, Apr, 2003
%

diju = 367*dmy(3) + dmy(1) - 712269 + fix(275*dmy(2)/9)- fix(7*(dmy(3)+fix((dmy(2)+9)/12))/4);

== matlab function kepler_basic_2021b/[MODE1] Propat : Kepler Differential Equation Integral(J2&J4)/Ephemerides Time1 ==
  data: hours input; dayf output; minutes input; seconds input
function dayf  = time_to_dayf(hours, minutes, seconds)
% [dayf] = time_to_dayf (hours, minutes, seconds)
%    The function time_to_dayf returns with the day elapesed
%    time in seconds
% inputs:
%   hours     
%       day hour (integer).
%   minutes
%       minutes (integer).
%   seconds
%       seconds and fraction of second
% outputs:
%   dayf
%       Day elapsed time in seconds. 
%
% Valdemir Carrara, Feb, 2009
%

dayf = seconds + 60*(minutes + 60*hours);

== matlab function kepler_basic_2021b/[MODE1] Propat : Kepler Differential Equation Integral(J2&J4)/Subsystem5/Keplerian Differential Equation ==
  data: kepel input; deltakep output
function deltakep  = delkep(kepel)
% [deltakep] = delkep (kep_el)
%	Function delkep calculates the rate of
%	variation of keplerian elements, considering only
%	J2 and J4.
%
% Input:
%	kep_el
% 		vector with the keplerian elements:
%		(1) - semimajor axis of the orbit in meters.
%		(2) - eccentricity.
%		(3) - inclination in radians.
%		(4) - right ascension of ascending node in radians.
%		(5) - argument of perigee in radians.
%		(6) - mean anomaly in radians.
%       Obs: 4,5 and 6 are not used
%
% Output:
%	deltakep
%		(1) = 0
%		(2) = 0
%		(3) = 0
%		(4) - variation rate of the right ascension of
%		      ascending node, in radians/second.
%		(5) - variation rate of the argument of perigee,
%			  in radians/second.
%		(6) - variation rate of the mean anomaly, in
%			  radians/second.
%
% Authors:
%	Valder M. de Medeiros  	september/81 	version 1.0
%	Valdemir Carrara 		july 2005		(C Version)
%   Valdemir Carrara            March/09        Matlab

EARTH_RADIUS	= 6378139.;				% Earth's radius in meters
EARTH_GRAVITY	= 3.9860064e+14;		% Earth's gravitational constant (m**3/s**2)
J_2 			=  1.0826268362e-3;		% = 484.16544e-6 * SQRT(5.e0)
J_4 			= -1.62336e-6;			% = -0.54112e-6 * 3e0

seix = kepel(1);
exce = kepel(2);
exc2 = exce*exce;
eta2 = 1. - exc2;
eta1 = sqrt(eta2);
teta = cos(kepel(3));
tet2 = teta*teta;
tet4 = tet2*tet2;
aux0 = sqrt(EARTH_GRAVITY/(seix*seix*seix));
plar = EARTH_RADIUS/(seix*eta2);
pla2 = plar*plar;
gam2 = 0.5*J_2*pla2;
gam4 = -0.375*J_4*pla2*pla2;

deltakep = [0, 0, 0, 0, 0, 0];

deltakep(4) = aux0*teta*(3.*gam2*(-1. + 0.125*gam2*(9.*eta2 + 12.*eta1 - ...
	   5. - (5.*eta2 + 36.*eta1 + 35.)*tet2)) + ...
	   1.25*gam4*(5. - 3.*eta2)*(3. - 7.*tet2));
deltakep(5) = aux0*(1.5*gam2*((5.*tet2 - 1.) + ...
	   0.0625*gam2*(25.*eta2 + 24.*eta1 - ...
	   35. + (90. - 192.*eta1 - 126.*eta2)*tet2 + ...
	   (385. + 360.*eta1 + 45.*eta2)*tet4)) + ...
	   0.3125*gam4*(21. - 9.*eta2 + (-270. + 126.*eta2)*tet2 + ...
	   (385. - 189.*eta2)*tet4));
deltakep(6) = aux0*(1. + eta1*(1.5*gam2*((3.*tet2 - 1.) + ...
	   0.0625*gam2*(16.*eta1 + 25.*eta2 - 15. + ...
	   (30. - 96.*eta1 - 90.*eta2)*tet2 + ...
	   (105. + 144.*eta1 + 25.*eta2)*tet4)) + ...
	   0.9375*gam4*exc2*(3. - 30.*tet2 + 35.*tet4)));

end

== matlab function kepler_basic_2021b/[MODE1] Propat : Kepler Differential Equation Integral(J2&J4)/MATLAB Function ==
  data: kepel input; statvec output
function statvec  = kepel_statvec (kepel)
%  [statvec] = kepel_statvec (kepel)
%	The function kepel_statvec transforms the keplerian
%	elements kepel into the corresponding state vector in
%	the same reference system.
%
% Input:
%	kepel
% 		vector containing the keplerian elements:
%		(1) - semimajor axis of the orbit in meters.
%		(2) - eccentricity.
%		(3) - inclinatsion in radians.
%		(4) - right ascension of ascending node in radians.
%		(5) - argument of perigee in radians.
%		(6) - mean anomaly in radians.
% Output:
%	statvec
%  		state vector in meters and meters/second.
%
% Authors:
%	Helio K. Kuga;
%	Valder M. Medeiros;
%	Valdemir Carrara		february/80		version 1.0
%	Valdemir Carrara		july 2005		(C version)
%   Valdemir Carrara            March/09        Matlab

EARTH_GRAVITY	= 3.9860064e+14;		% Earth's gravitational constant (m**3/s**2)

a    = kepel(1);	% semi-major axis
exc  = kepel(2);	% eccentricity

c1   = sqrt(1. - exc*exc);

%     rotation matrix

orb2iner = rotmaz(-kepel(4))*rotmax(-kepel(3))*rotmaz(-kepel(5));

%     Kepler's equation

E    = kepler(kepel(6), exc);

sE   = sin(E);
cE   = cos(E);
c3   = sqrt(EARTH_GRAVITY/a)/(1. - exc*cE);

%     state vector

statvec = [[a*(cE - exc), a*c1*sE, 0]*orb2iner', [-c3*sE, c1*c3*cE, 0]*orb2iner'];

end

function [rot_mat] = rotmax (angle)
% [rot_mat] = rotmax (angle)
%   To obtain the rotation matrix around the X axis given the
%   rotation angle.
% inputs:
%   angle
%       rotation angle, in radians.
% outputs:
%   rot_mat
%       rotation matrix (3, 3)
%

% Valdemir Carrara, Sep, 1998

coan    =  cos(angle);
sian    =  sin(angle);

rot_mat =  [1, 0, 0; 0, coan, sian; 0, -sian, coan];

end

function [rot_mat] = rotmay (angle)
% [rot_mat] = rotmay (angle)
%   To obtain the rotation matrix around the Y axis given the
%   rotation angle.
% inputs:
%   angle
%       rotation angle, in radians.
% outputs:
%   rot_mat
%       rotation matrix (3, 3)
%

% Valdemir Carrara, Sep, 1998


coan    =  cos(angle);
sian    =  sin(angle);

rot_mat =  [coan, 0, -sian; 0, 1, 0; sian, 0, coan];

end

function [rot_mat] = rotmaz (angle)
% [rot_mat] = rotmaz (angle)
%   To obtain the rotation matrix around the Z axis given the
%   rotation angle.
% inputs:
%   angle
%       rotation angle, in radians.
% outputs:
%   rot_mat
%       rotation matrix (3, 3)
%

% Valdemir Carrara, Sep, 1998

coan    =  cos(angle);
sian    =  sin(angle);

rot_mat =  [coan, sian, 0; -sian, coan, 0; 0, 0, 1];
end

function [eccentric] = kepler (mean_anomaly, eccentricity)
% [eccentric] = kepler (mean_anomaly, eccentricity)
%	The subroutine kepler finds a solution to the
%	kepler's equation.
%
% Input:
%	mean_anomaly
%		mean anomaly in radians.
%	eccentricity
%		eccentricity.
%
% Output:
%	eccentric
%		eccentric anomaly in radians.
%
% Authors:
%	Valder M. de Medeiros		june/81		version 2.0
%	Valdemir Carrara			july 2005	(C version)
%   Valdemir Carrara            March/09        Matlab

exc2    = eccentricity*eccentricity;
am1     = mod (mean_anomaly, 2*pi);
am2     = am1 + am1;
am3     = am1 + am2;
shoot   = am1 + eccentricity*(1. - 0.125*exc2)*sin(am1) + ...
		0.5*exc2*(sin(am2) + 0.75*eccentricity*sin(am3));
shoot   = mod (shoot, 2*pi);

e1      = 1.0;
ic      = 0;

while ((abs(e1) > 1.e-12) && (ic <= 10)) 
	e1    = (shoot - am1 - eccentricity*sin(shoot)) / ...
			(1.0 - eccentricity*cos(shoot));
    shoot = shoot - e1;
    ic    = ic + 1;
end

if (ic >= 10)
    disp ('warning ** subroutine kepler did not converge in 10 iterations');
end

eccentric = shoot;


end

== matlab function kepler_basic_2021b/[MODE2] Propat : Kepler to Statevec using Only Mean Anomaly/MATLAB Function2 ==
  data: kepel input; statvec output
function statvec  = kepel_statvec (kepel)
%  [statvec] = kepel_statvec (kepel)
%	The function kepel_statvec transforms the keplerian
%	elements kepel into the corresponding state vector in
%	the same reference system.
%
% Input:
%	kepel
% 		vector containing the keplerian elements:
%		(1) - semimajor axis of the orbit in meters.
%		(2) - eccentricity.
%		(3) - inclinatsion in radians.
%		(4) - right ascension of ascending node in radians.
%		(5) - argument of perigee in radians.
%		(6) - mean anomaly in radians.
% Output:
%	statvec
%  		state vector in meters and meters/second.
%
% Authors:
%	Helio K. Kuga;
%	Valder M. Medeiros;
%	Valdemir Carrara		february/80		version 1.0
%	Valdemir Carrara		july 2005		(C version)
%   Valdemir Carrara            March/09        Matlab

EARTH_GRAVITY	= 3.9860064e+14;		% Earth's gravitational constant (m**3/s**2)

a    = kepel(1);	% semi-major axis
exc  = kepel(2);	% eccentricity

c1   = sqrt(1. - exc*exc);

%     rotation matrix

orb2iner = rotmaz(-kepel(4))*rotmax(-kepel(3))*rotmaz(-kepel(5));

%     Kepler's equation

E    = kepler(kepel(6), exc);

sE   = sin(E);
cE   = cos(E);
c3   = sqrt(EARTH_GRAVITY/a)/(1. - exc*cE);

%     state vector

statvec = [[a*(cE - exc), a*c1*sE, 0]*orb2iner', [-c3*sE, c1*c3*cE, 0]*orb2iner'];

end

function [rot_mat] = rotmax (angle)
% [rot_mat] = rotmax (angle)
%   To obtain the rotation matrix around the X axis given the
%   rotation angle.
% inputs:
%   angle
%       rotation angle, in radians.
% outputs:
%   rot_mat
%       rotation matrix (3, 3)
%

% Valdemir Carrara, Sep, 1998

coan    =  cos(angle);
sian    =  sin(angle);

rot_mat =  [1, 0, 0; 0, coan, sian; 0, -sian, coan];

end

function [rot_mat] = rotmay (angle)
% [rot_mat] = rotmay (angle)
%   To obtain the rotation matrix around the Y axis given the
%   rotation angle.
% inputs:
%   angle
%       rotation angle, in radians.
% outputs:
%   rot_mat
%       rotation matrix (3, 3)
%

% Valdemir Carrara, Sep, 1998


coan    =  cos(angle);
sian    =  sin(angle);

rot_mat =  [coan, 0, -sian; 0, 1, 0; sian, 0, coan];

end

function [rot_mat] = rotmaz (angle)
% [rot_mat] = rotmaz (angle)
%   To obtain the rotation matrix around the Z axis given the
%   rotation angle.
% inputs:
%   angle
%       rotation angle, in radians.
% outputs:
%   rot_mat
%       rotation matrix (3, 3)
%

% Valdemir Carrara, Sep, 1998

coan    =  cos(angle);
sian    =  sin(angle);

rot_mat =  [coan, sian, 0; -sian, coan, 0; 0, 0, 1];
end

function [eccentric] = kepler (mean_anomaly, eccentricity)
% [eccentric] = kepler (mean_anomaly, eccentricity)
%	The subroutine kepler finds a solution to the
%	kepler's equation.
%
% Input:
%	mean_anomaly
%		mean anomaly in radians.
%	eccentricity
%		eccentricity.
%
% Output:
%	eccentric
%		eccentric anomaly in radians.
%
% Authors:
%	Valder M. de Medeiros		june/81		version 2.0
%	Valdemir Carrara			july 2005	(C version)
%   Valdemir Carrara            March/09        Matlab

exc2    = eccentricity*eccentricity;
am1     = mod (mean_anomaly, 2*pi);
am2     = am1 + am1;
am3     = am1 + am2;
shoot   = am1 + eccentricity*(1. - 0.125*exc2)*sin(am1) + ...
		0.5*exc2*(sin(am2) + 0.75*eccentricity*sin(am3));
shoot   = mod (shoot, 2*pi);

e1      = 1.0;
ic      = 0;

while ((abs(e1) > 1.e-12) && (ic <= 10)) 
	e1    = (shoot - am1 - eccentricity*sin(shoot)) / ...
			(1.0 - eccentricity*cos(shoot));
    shoot = shoot - e1;
    ic    = ic + 1;
end

if (ic >= 10)
    disp ('warning ** subroutine kepler did not converge in 10 iterations');
end

eccentric = shoot;


end

== matlab function kepler_basic_2021b/[Mode3] Basic Kepler Propagate/Kepler Propagate ==
  data: initial_condition input; dfdt output
function dfdt  = eq_propagate(initial_condition)
% Lectures_TwoBodyProblem.pdf
% 우주시스템입문 - 도미타 노부유키 eq(7.8) p136
% https://en.wikipedia.org/wiki/Standard_gravitational_parameter
u  = 3.9865*10^14; % earth gravitional parameter
Re = 6378137;      % earth radius [m]

dfdt = zeros(size(initial_condition));

% x=x
% x1=dx/dt
% dx1/dt = d^2(x)/dt

x1 = initial_condition(4); % x1 = dx/dt
y1 = initial_condition(5); % y1 = dy/dt
z1 = initial_condition(6); % z1 = dz/dt
x  = initial_condition(1); % x
y  = initial_condition(2); % y
z  = initial_condition(3); % z

r=sqrt(x^2+y^2+z^2);

% % %   Keplar Motion Equatnion
% % %  => r_dd + u/(r^3)r_ = 0 => r_dd = -u/(r^3)r_
dfdt(1) = x1;
dfdt(2) = y1;
dfdt(3) = z1;
dfdt(4) = -u*x/r^3;
dfdt(5) = -u*y/r^3;
dfdt(6) = -u*z/r^3;

end

== matlab function kepler_basic_2021b/[MODE2] Propat : Kepler to Statevec using Only Mean Anomaly/MATLAB Function1 ==
  data: kep_init input; kep_modified output
function kep_modified = fcn(kep_init)

persistent f_flg
persistent kep0
persistent mean_anomaly

if isempty(f_flg)
    kep0 = kep_init;
    mean_anomaly = kep_init(6);
    f_flg = 1;
else
    mean_anomaly = mean_anomaly + 0.001;
end

    kep_modified = [kep0(1),kep0(2),kep0(3),kep0(4),kep0(5),mean_anomaly];

end
